simulink model "problem2"  (Simulink 7.7)
settings: Solver=ode3  StartTime=0.0  StopTime=600  FixedStep=.5  RelTol=1e-3
settings Model: Creator=Ed  LastModifiedBy=Ed

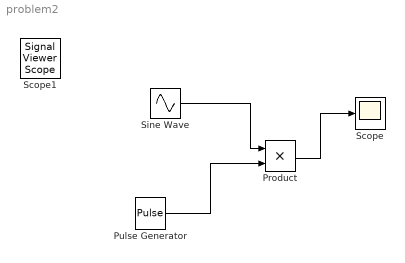
== system problem2 ==
  Product : Product  RndMeth=Zero
  Pulse Generator : DiscretePulseGenerator  PulseType=Time based  Period=12  PulseWidth=50
  Scope : Scope
  Sine Wave : Sin  Frequency=0.0104719755  SampleTime=0
  Scope1 : SignalViewerScope  IOType=viewer  RefreshTime=0.035000
  wires:
  Sine Wave/1 -> Product/1
  Pulse Generator/1 -> Product/2
  Product/1 -> Scope/1
